simulink model "aeb_ut"  (Simulink 8.1)
settings: Solver=FixedStepDiscrete  StartTime=0.0  StopTime=10  FixedStep=5e-3  RelTol=1e-3
PostLoadFcn:
  | , if any(exist('dsrtsu_mdlpostloadfcn', 'file') == [2, 3, 6]), try dsrtsu_mdlpostloadfcn('Execute', bdroot); catch fprintf('Error in PostLoadFcn (dsrtsu_mdlpostloadfcn) for model "%s":\n %s\n', bdroot, lasterr); end, end,
undefined symbols (not defined in the file or in its folder): VJUD_AEBActionReq_flg, VJUD_AEBAutoBraking_flg, VJUD_AEBDeactivationReq_flg, VJUD_AEBEnableReq_flg, VJUD_AEBOperational_flg, VJUD_AEBReturnOperational_flg, VJUD_AEBSpeedInRange_flg
libraries: siltestlib x23, aeb x1, simulink x1
settings Model: DSRTSU_INTERNAL_RTI_VER=450  DSRTSU_INTERNAL_RTI_TYPE=rti1401  RTICANMMDATA=struct('GeneralSetupData',struct('modelroot','D:\Soichi\SVNDATA\IDIADA_ADAS\trunk\AdasDragon\software\sw_development\arch\app\aeb','generalsettings',struct('filesettings',struct('destfolder',struct('Name','RTICANMM_FILES','Check',1),'buildfolder',struct('Name','.','Check',1),'AbsDestfolder',struct('Name','D:\Soichi\SVNDATA\IDIADA_ADAS\trunk\AdasDragon\software\sw_development\arch\app\aeb\RTICANMM_FILES'),'AbsBuildfolder',struct('Name','D:\Soichi\SVNDATA\IDIADA_ADAS\trunk\AdasDragon\software\sw_development\arch\app\aeb'))),'options',struct('addpaths',1,'rmpaths',1,'addtrcexclusion',logical(1),'cannavigator',struct('checkmonitoring',0),'show_usrtrc',0,'use_usrtrc',0),'advanced',struct('options',[1 1 1 1 1 1 1 1 1 1 1 1 1 1 1 1 1 1 1 1 1 1 1 1 1 1 1 1 1 1 1 1 1 1 1 1 1 1 1 1 1 1 1 1 1 1 1 1 1 1 1 1 1 1 1 1 1 1 1 1 1 1 1 1 1 1 1 1 1 1 1 1 1 1 1 1 1 1 1 1 1 1 1 1 1 1 1 1 1 1 1 1 1 1 1 1 1 1 1 1]),'MPSetup',{{}},'modelname','aeb_ut','block','aeb_ut'))  DSRTSU_INTERNAL_RTIFPGA=40  Creator=AT015411  LastModifiedBy=AT015411  BufferReuse=off
settings DataIOCC: SignalLoggingSaveFormat=Dataset
settings OptimizationCC: BlockReduction=off  OptimizeBlockIOStorage=off  BufferReuse=off  ExpressionFolding=off  ExpressionDepthLimit=128  LocalBlockOutputs=off
settings DebuggingCC: FcnCallInpInsideContextMsg=EnableAllAsError
settings HardwareCC: ProdIntDivRoundTo=Zero  ProdEndianess=BigEndian  ProdHWDeviceType=Generic->Custom  TargetIntDivRoundTo=Zero  TargetEndianess=BigEndian  TargetHWDeviceType=Generic->Custom
settings RTWCC: SystemTargetFile=rti1005.tlc  MakeCommand=make_rti  TemplateMakefile=rti1005.tmf  Description=dSPACE DS1005 Hardware Platform  ProcessScript=rti1005_make_rtw_hook
settings STFCustomTargetCC: CodeReplacementLibrary=ANSI_C  ParMdlRefBuildCompliant=on  GeneratePreprocessorConditionals=Disable all  MatFileLogging=on  SystemTargetFile=rti1005.tlc
settings GRTTargetCC: CompOptLevelCompliant=off  ConcurrentExecutionCompliant=off  ExtModeMexFile=noextcomm
settings CustomProperty: DataType=RTWOptions_EnumType_D__Program Files_dSPACE RCPHIL 2014-B_MATLAB_RTI_RTI1401_TLC_rti1005_1InitialSimState  Value=RUN
settings EnumStrPairs: String=RUN

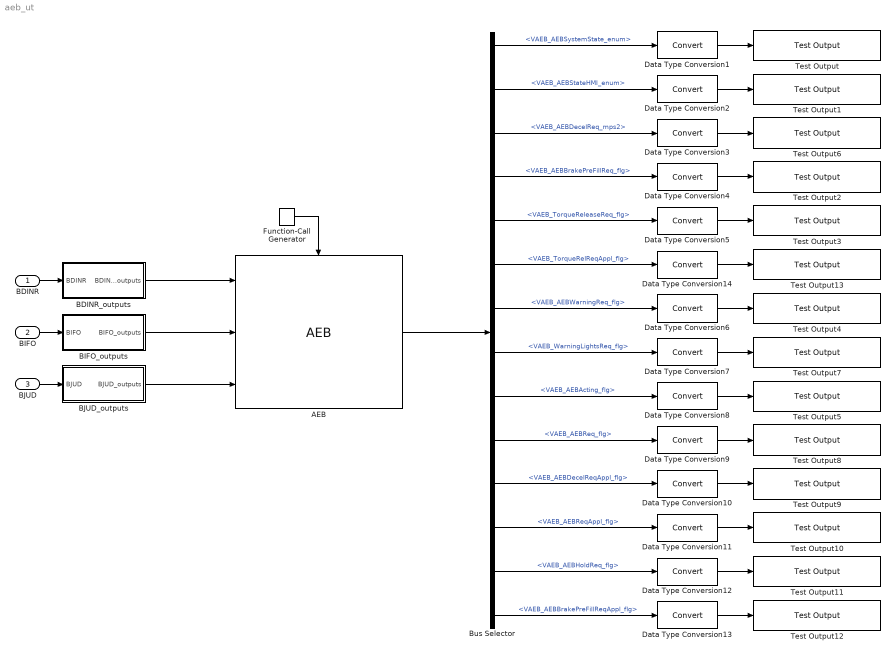
== system aeb_ut ==
  BDINR : Inport  OutDataTypeStr=Bus: BDINR_outputs
  BIFO : Inport  Port=2  OutDataTypeStr=Bus: BIFO_outputs
  BJUD : Inport  Port=3  OutDataTypeStr=Bus: BJUD_outputs
  AEB : aeb/AEB
  BDINR_outputs : Subsystem
  BIFO_outputs : Subsystem
  BJUD_outputs : Subsystem
  Bus Selector : BusSelector  OutputSignals=VAEB_AEBSystemState_enum,VAEB_AEBStateHMI_enum,VAEB_AEBDecelReq_mps2,VAEB_AEBBrakePreFillReq_flg,VAEB_TorqueReleaseReq_flg,VAEB_TorqueRelReqAppl_flg,VAEB_AEBWarningReq_flg,VAEB_WarningLightsReq_flg,VAEB_AEBActing_flg,VAEB_AEBReq_flg,VAEB_AEBDecelReqAppl_flg,VAEB_AEBReqAppl_flg,VAEB_AEBHoldReq_flg,VAEB_AEBBrakePreFillReqAppl_flg
  Data Type Conversion{1..14} (14 alike) : DataTypeConversion
  Function-Call Generator : simulink/Ports & Subsystems/Function-Call Generator  sample_time=5e-3  numberOfIterations=1
  Test Output : siltestlib/Test Output  varname=VAEB_AEBSystemState_enum  sampletime=-1
  Test Output1 : siltestlib/Test Output  varname=VAEB_AEBStateHMI_enum  sampletime=-1
  Test Output10 : siltestlib/Test Output  varname=VAEB_AEBReqAppl_flg  sampletime=-1
  Test Output11 : siltestlib/Test Output  varname=VAEB_AEBHoldReq_flg  sampletime=-1
  Test Output12 : siltestlib/Test Output  varname=VAEB_AEBBrakePreFillReqAppl_flg  sampletime=-1
  Test Output13 : siltestlib/Test Output  varname=VAEB_TorqueRelReqAppl_flg  sampletime=-1
  Test Output2 : siltestlib/Test Output  varname=VAEB_AEBBrakePreFillReq_flg  sampletime=-1
  Test Output3 : siltestlib/Test Output  varname=VAEB_TorqueReleaseReq_flg  sampletime=-1
  Test Output4 : siltestlib/Test Output  varname=VAEB_AEBWarningReq_flg  sampletime=-1
  Test Output5 : siltestlib/Test Output  varname=VAEB_AEBActing_flg  sampletime=-1
  Test Output6 : siltestlib/Test Output  varname=VAEB_AEBDecelReq_mps2  sampletime=-1
  Test Output7 : siltestlib/Test Output  varname=VAEB_WarningLightsReq_flg  sampletime=-1
  Test Output8 : siltestlib/Test Output  varname=VAEB_AEBReq_flg  sampletime=-1
  Test Output9 : siltestlib/Test Output  varname=VAEB_AEBDecelReqAppl_flg  sampletime=-1
  wires:
  BDINR_outputs/1(BDINR_outputs) -> AEB/1
  BIFO_outputs/1(BIFO_outputs) -> AEB/2
  BJUD_outputs/1(BJUD_outputs) -> AEB/3
  Bus Selector/1 -> Data Type Conversion1/1  "<VAEB_AEBSystemState_enum>"
  Data Type Conversion1/1 -> Test Output/1
  Bus Selector/2 -> Data Type Conversion2/1  "<VAEB_AEBStateHMI_enum>"
  Data Type Conversion2/1 -> Test Output1/1
  Bus Selector/3 -> Data Type Conversion3/1  "<VAEB_AEBDecelReq_mps2>"
  Data Type Conversion4/1 -> Test Output2/1
  Bus Selector/4 -> Data Type Conversion4/1  "<VAEB_AEBBrakePreFillReq_flg>"
  Data Type Conversion5/1 -> Test Output3/1
  Bus Selector/5 -> Data Type Conversion5/1  "<VAEB_TorqueReleaseReq_flg>"
  Data Type Conversion6/1 -> Test Output4/1
  Bus Selector/7 -> Data Type Conversion6/1  "<VAEB_AEBWarningReq_flg>"
  Data Type Conversion8/1 -> Test Output5/1
  AEB/1 -> Bus Selector/1
  Bus Selector/8 -> Data Type Conversion7/1  "<VAEB_WarningLightsReq_flg>"
  Data Type Conversion3/1 -> Test Output6/1
  Bus Selector/9 -> Data Type Conversion8/1  "<VAEB_AEBActing_flg>"
  Data Type Conversion7/1 -> Test Output7/1
  Function-Call Generator/1 -> AEB/Trigger
  BDINR/1 -> BDINR_outputs/1(BDINR)
  BJUD/1 -> BJUD_outputs/1(BJUD)
  BIFO/1 -> BIFO_outputs/1(BIFO)
  Data Type Conversion9/1 -> Test Output8/1
  Bus Selector/10 -> Data Type Conversion9/1  "<VAEB_AEBReq_flg>"
  Data Type Conversion10/1 -> Test Output9/1
  Bus Selector/11 -> Data Type Conversion10/1  "<VAEB_AEBDecelReqAppl_flg>"
  Data Type Conversion11/1 -> Test Output10/1
  Bus Selector/12 -> Data Type Conversion11/1  "<VAEB_AEBReqAppl_flg>"
  Data Type Conversion12/1 -> Test Output11/1
  Bus Selector/13 -> Data Type Conversion12/1  "<VAEB_AEBHoldReq_flg>"
  Data Type Conversion13/1 -> Test Output12/1
  Bus Selector/14 -> Data Type Conversion13/1  "<VAEB_AEBBrakePreFillReqAppl_flg>"
  Data Type Conversion14/1 -> Test Output13/1
  Bus Selector/6 -> Data Type Conversion14/1  "<VAEB_TorqueRelReqAppl_flg>"

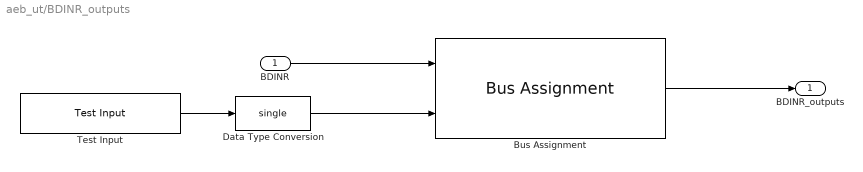
== system aeb_ut/BDINR_outputs ==
  BDINR : Inport  OutDataTypeStr=Bus: BDINR_outputs
  Bus Assignment : BusAssignment  AssignedSignals=VDINR_VehSpd_mps
  Data Type Conversion : DataTypeConversion  OutDataTypeStr=single
  Test Input : siltestlib/Test Input  varname=VDINR_VehSpd_mps  sampletime=-1
  BDINR_outputs : Outport  OutDataTypeStr=Bus: BDINR_outputs
  wires:
  Bus Assignment/1 -> BDINR_outputs/1
  BDINR/1 -> Bus Assignment/1
  Test Input/1 -> Data Type Conversion/1
  Data Type Conversion/1 -> Bus Assignment/2

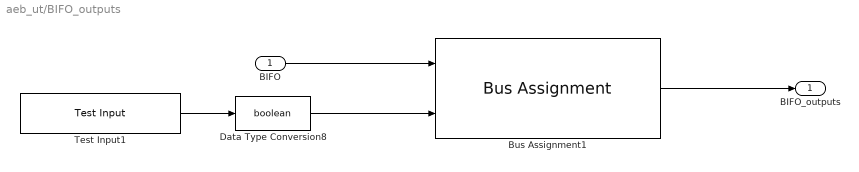
== system aeb_ut/BIFO_outputs ==
  BIFO : Inport  OutDataTypeStr=Bus: BIFO_outputs
  Bus Assignment1 : BusAssignment  AssignedSignals=VIFO_BrakePedalPressed_flg
  Data Type Conversion8 : DataTypeConversion  OutDataTypeStr=boolean
  Test Input1 : siltestlib/Test Input  varname=VIFO_BrakePedalPressed_flg  sampletime=-1
  BIFO_outputs : Outport  OutDataTypeStr=Bus: BIFO_outputs
  wires:
  BIFO/1 -> Bus Assignment1/1
  Bus Assignment1/1 -> BIFO_outputs/1
  Test Input1/1 -> Data Type Conversion8/1
  Data Type Conversion8/1 -> Bus Assignment1/2

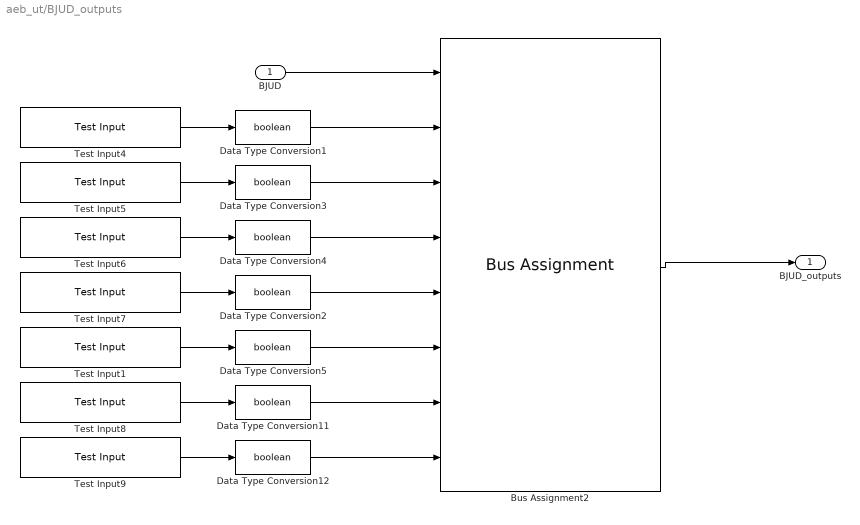
== system aeb_ut/BJUD_outputs ==
  BJUD : Inport  OutDataTypeStr=Bus: BJUD_outputs
  Bus Assignment2 : BusAssignment  AssignedSignals=VJUD_AEBEnableReq_flg,VJUD_AEBSpeedInRange_flg,VJUD_AEBOperational_flg,VJUD_AEBActionReq_flg,VJUD_AEBReturnOperational_flg,VJUD_AEBAutoBraking_flg,VJUD_AEBDeactivationReq_flg
  Data Type Conversion{1..5,11..12} (7 alike) : DataTypeConversion  OutDataTypeStr=boolean
  Test Input1 : siltestlib/Test Input  varname=VJUD_AEBReturnOperational_flg  sampletime=-1
  Test Input4 : siltestlib/Test Input  varname=VJUD_AEBEnableReq_flg  sampletime=-1
  Test Input5 : siltestlib/Test Input  varname=VJUD_AEBSpeedInRange_flg  sampletime=-1
  Test Input6 : siltestlib/Test Input  varname=VJUD_AEBOperational_flg  sampletime=-1
  Test Input7 : siltestlib/Test Input  varname=VJUD_AEBActionReq_flg  sampletime=-1
  Test Input8 : siltestlib/Test Input  varname=VJUD_AEBAutoBraking_flg  sampletime=-1
  Test Input9 : siltestlib/Test Input  varname=VJUD_AEBDeactivationReq_flg  sampletime=-1
  BJUD_outputs : Outport  OutDataTypeStr=Bus: BJUD_outputs
  wires:
  BJUD/1 -> Bus Assignment2/1
  Bus Assignment2/1 -> BJUD_outputs/1
  Test Input4/1 -> Data Type Conversion1/1
  Data Type Conversion1/1 -> Bus Assignment2/2
  Test Input5/1 -> Data Type Conversion3/1
  Data Type Conversion3/1 -> Bus Assignment2/3
  Test Input6/1 -> Data Type Conversion4/1
  Data Type Conversion4/1 -> Bus Assignment2/4
  Test Input7/1 -> Data Type Conversion2/1
  Data Type Conversion2/1 -> Bus Assignment2/5
  Test Input8/1 -> Data Type Conversion11/1
  Data Type Conversion11/1 -> Bus Assignment2/7
  Test Input9/1 -> Data Type Conversion12/1
  Data Type Conversion12/1 -> Bus Assignment2/8
  Test Input1/1 -> Data Type Conversion5/1
  Data Type Conversion5/1 -> Bus Assignment2/6
